simulink model "Practica5_Simulink"  (R2024a)
settings: Solver=VariableStepAuto  StartTime=0.0  StopTime=0.001  MaxStep=0.01  RelTol=1e-6
InitFcn:
  | C=0.1e-6;
  | R=100;
  | L=8e-3;
settings Model: Creator=Manuel  LastModifiedBy=Manuel

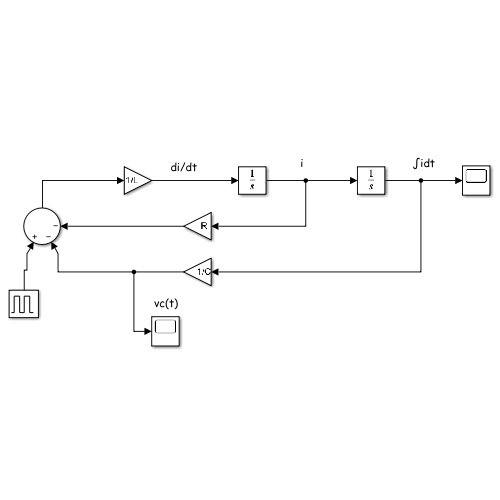
[thumbnail: Simulink's stored preview of the top-level diagram]
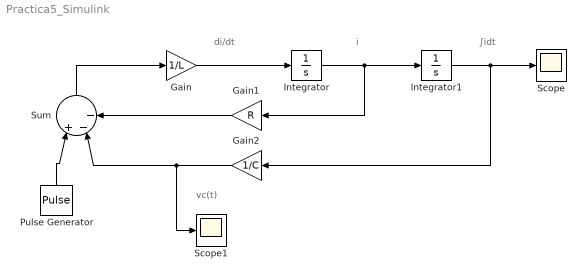
== system Practica5_Simulink ==
  note: ∫idt
  note: i
  note: di/dt
  note: vc(t)
  Gain : Gain  Gain=1/L
  Gain1 : Gain  Gain=R
  Gain2 : Gain  Gain=1/C
  Integrator : Integrator
  Integrator1 : Integrator
  Pulse Generator : DiscretePulseGenerator  PulseType=Time based  Amplitude=12  Period=0.002  PulseWidth=50
  Scope : Scope
  Scope1 : Scope
  Sum : Sum  Inputs=|+--
  wires:
  Integrator/1 -> Gain1/1, Integrator1/1
  Integrator1/1 -> Gain2/1, Scope/1
  Gain/1 -> Integrator/1
  Gain1/1 -> Sum/3
  Gain2/1 -> Scope1/1, Sum/2
  Pulse Generator/1 -> Sum/1
  Sum/1 -> Gain/1
